simulink model "System_2"  (R2020a)
settings: Solver=FixedStepAuto  StartTime=0.0  StopTime=10.0  FixedStep=1  RelTol=1e-3
settings Model: Creator=NIKITA  LastModifiedBy=NIKITA
settings DataIOCC: SaveOutput=off  SaveTime=off

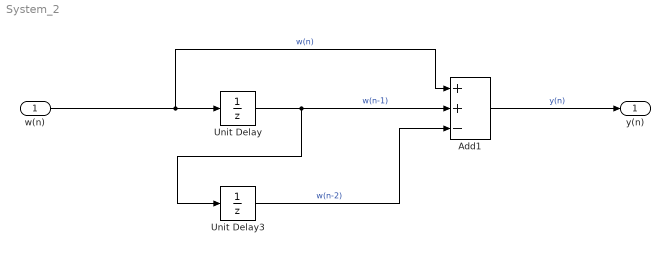
== system System_2 ==
  w(n) : Inport  OutDataTypeStr=double  PortDimensions=[1 1]  SampleTime=[1,0]
  Add1 : Sum  Inputs=++-
  Unit Delay : UnitDelay  SampleTime=-1  HasFrameUpgradeWarning=on
  Unit Delay3 : UnitDelay  SampleTime=-1  HasFrameUpgradeWarning=on
  y(n) : Outport  OutDataTypeStr=double  PortDimensions=[1 1]  SampleTime=[1,0]
  wires:
  w(n)/1 -> Unit Delay/1, Add1/1  "w(n)"
  Unit Delay3/1 -> Add1/3  "w(n-2)"
  Unit Delay/1 -> Unit Delay3/1, Add1/2  "w(n-1)"
  Add1/1 -> y(n)/1  "y(n)"
